simulink model "Buck_model"  (R2024a)
settings: Solver=odeN  StartTime=0.0  StopTime=35  MaxStep=Ts_motor  RelTol=1e-3  EnableMultiTasking=on
InitFcn:
  | load bldcData
model workspace (MAT data in the model file):
  encoderResolution = 2000
  hallOffset = '0.5'
  indexOffset = 850
  polePairs = '4'
undefined symbols (not defined in the file or in its folder): DiscIntNeverNeededParam, Hecate_speed, Ts_motor
libraries: nesl_utility x25, fl_lib x24, ee_lib x7, batteryecm_lib x1, spsPWMGeneratorDCDCLib x1, slpidlib x1, simulink x1
(part 2 of 2)

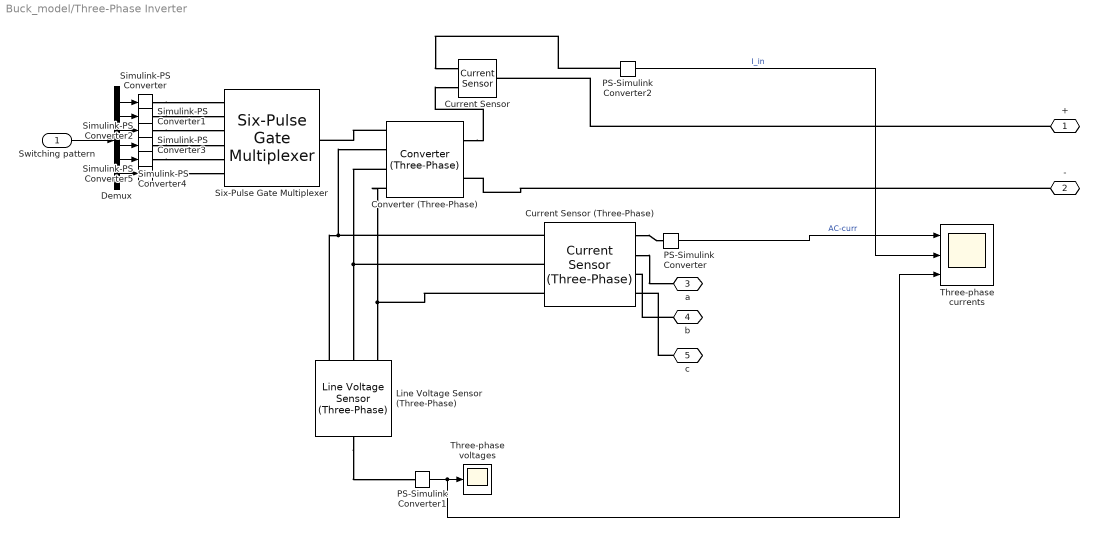
== system Buck_model/Three-Phase Inverter ==
  Switching pattern : Inport
  Converter (Three-Phase) : ee_lib/Semiconductors & Converters/Converters/Converter (Three-Phase)  port_option=ee.enum.threePhasePort.expanded  fidelity_option=ee.enum.converters.fidelity.detailed  device_type=ee.enum.converters.switchingdevice.mosfet  K=0  Vf=0.8 V  Ron=0.1 Ohm  Rds=0.001 Ohm  Goff=0.001 1/Ohm  Vgt=1 V  Vgt_off=-1 V  Ih=1 A  Vth=0.5 V  diode_param=ee.enum.converters.protectiondiode.nodynamics  diode_Vf=0.7 V  diode_Ron=0.001 Ohm  diode_Goff=1e-5 1/Ohm  diode_C=50 nF  diode_iRM=-235 A  diode_iF=300 A  diode_idot=-50 A/us  diode_trr_param=ee.enum.converters.diodetrr.trr_factor  diode_trr_factor=3  diode_trr=15 us  diode_Qrr=1500 s*uA  snubber_type=ee.enum.converters.snubber.include  Cs=1e-7 F  Rs=0.1 Ohm
      settings: InternalSimscapePortConfiguration="{\"Bottom\":[],\"Left\":[{\"id\":\"G\",\"label\":\"G\",\"type\":\"foundation.electrical.twelve_phase\"},{\"id\":\"a\",\"label\":\"a\",\"type\":\"foundation.electrical.electrical\"},{\"id\":\"b\",\"label\":\"b\",\"type\":\"foundation.electrical.electrical\"},{\"id\":\"c\",\"label\":\"c\",\"type\":\"foundation.electrical.electrical\"}],\"Right\":[{\"id\":\"p\",\"label\":\"+\",\"type\":\"foundation.electrical.electrical\"},{\"id\":\"n\",\"label\":\"-\",\"type\":\"foundation.electrical.electrical\"}],\"Top\":[]}"
  Current Sensor : fl_lib/Electrical/Electrical Sensors/Current Sensor
  Current Sensor (Three-Phase) : ee_lib/Sensors & Transducers/Current Sensor (Three-Phase)
      settings: InternalSimscapePortConfiguration="{\"Bottom\":[],\"Left\":[{\"id\":\"a1\",\"label\":\"a1\",\"type\":\"foundation.electrical.electrical\"},{\"id\":\"b1\",\"label\":\"b1\",\"type\":\"foundation.electrical.electrical\"},{\"id\":\"c1\",\"label\":\"c1\",\"type\":\"foundation.electrical.electrical\"}],\"Right\":[{\"id\":\"I_output\",\"label\":\"I\",\"type\":\"output\"},{\"id\":\"a2\",\"label\":\"a2\",\"type\":\"foundation.electrical.electrical\"},{\"id\":\"b2\",\"label\":\"b2\",\"type\":\"foundation.electrical.electrical\"},{\"id\":\"c2\",\"label\":\"c2\",\"type\":\"foundation.electrical.electrical\"}],\"Top\":[]}"
  Demux : Demux  Outputs=6
  Line Voltage Sensor (Three-Phase) : ee_lib/Sensors & Transducers/Line Voltage Sensor (Three-Phase)
      settings: InternalSimscapePortConfiguration="{\"Bottom\":[],\"Left\":[{\"id\":\"a\",\"label\":\"a\",\"type\":\"foundation.electrical.electrical\"},{\"id\":\"b\",\"label\":\"b\",\"type\":\"foundation.electrical.electrical\"},{\"id\":\"c\",\"label\":\"c\",\"type\":\"foundation.electrical.electrical\"}],\"Right\":[{\"id\":\"V_output\",\"label\":\"V\",\"type\":\"output\"}],\"Top\":[]}"
  PS-Simulink Converter : nesl_utility/PS-Simulink Converter  PhysicalDomain=network_engine_domain  SubClassName=ps_output  LeftPortType=input  RightPortType=output  PseudoPeriodic=off  Frequencies=[]  VectorFormat=1-D array  Unit=1  AffineConversion=off
  PS-Simulink Converter1 : nesl_utility/PS-Simulink Converter  PhysicalDomain=network_engine_domain  SubClassName=ps_output  LeftPortType=input  RightPortType=output  PseudoPeriodic=off  Frequencies=[]  VectorFormat=1-D array  Unit=1  AffineConversion=off
  PS-Simulink Converter2 : nesl_utility/PS-Simulink Converter  PhysicalDomain=network_engine_domain  SubClassName=ps_output  LeftPortType=input  RightPortType=output  PseudoPeriodic=off  Frequencies=[]  VectorFormat=1-D array  Unit=1  AffineConversion=off
  Simulink-PS Converter{,1..5} (6 alike) : nesl_utility/Simulink-PS Converter  PhysicalDomain=network_engine_domain  SubClassName=ps_input  LeftPortType=input  RightPortType=output  PseudoPeriodic=off  Frequencies=[]  NoiseDistribution=none  NoiseParameters=[]  Unit=1  AffineConversion=off  FilteringAndDerivatives=provide  SimscapeFilterOrder=1  InputFilterTimeConstant=0.001  UdotUserProvided=0
  Six-Pulse Gate Multiplexer : ee_lib/Semiconductors & Converters/Converters/Six-Pulse Gate Multiplexer  port_option=ee.enum.controlport.ps
  Three-phase currents : Scope  NumInputPorts=3
  Three-phase voltages : Scope
  + : PMIOPort  Side=Left
  - : PMIOPort  Port=2  Side=Left
  a : PMIOPort  Port=3  Side=Right
  b : PMIOPort  Port=4  Side=Right
  c : PMIOPort  Port=5  Side=Right
  wires:
  PS-Simulink Converter1/1 -> Three-phase currents/3, Three-phase voltages/1
  PS-Simulink Converter/1 -> Three-phase currents/1  "AC-curr"
  Switching pattern/1 -> Demux/1
  Demux/1 -> Simulink-PS Converter/1
  Demux/2 -> Simulink-PS Converter1/1
  Demux/3 -> Simulink-PS Converter2/1
  Demux/4 -> Simulink-PS Converter3/1
  Demux/5 -> Simulink-PS Converter4/1
  Demux/6 -> Simulink-PS Converter5/1
  PS-Simulink Converter2/1 -> Three-phase currents/2  "I_in"
  connections:
  Current Sensor (Three-Phase)/RConn1 -- PS-Simulink Converter/LConn1
  Simulink-PS Converter/RConn1 -- Six-Pulse Gate Multiplexer/LConn1
  Simulink-PS Converter1/RConn1 -- Six-Pulse Gate Multiplexer/LConn2
  Simulink-PS Converter2/RConn1 -- Six-Pulse Gate Multiplexer/LConn3
  Simulink-PS Converter3/RConn1 -- Six-Pulse Gate Multiplexer/LConn4
  Simulink-PS Converter4/RConn1 -- Six-Pulse Gate Multiplexer/LConn5
  Simulink-PS Converter5/RConn1 -- Six-Pulse Gate Multiplexer/LConn6
  Converter (Three-Phase)/LConn1 -- Six-Pulse Gate Multiplexer/RConn1
  Line Voltage Sensor (Three-Phase)/LConn1 -- Current Sensor (Three-Phase)/LConn1 -- Converter (Three-Phase)/LConn2
  Line Voltage Sensor (Three-Phase)/RConn1 -- PS-Simulink Converter1/LConn1
  Converter (Three-Phase)/LConn3 -- Current Sensor (Three-Phase)/LConn2 -- Line Voltage Sensor (Three-Phase)/LConn2
  Converter (Three-Phase)/LConn4 -- Current Sensor (Three-Phase)/LConn3 -- Line Voltage Sensor (Three-Phase)/LConn3
  Current Sensor (Three-Phase)/RConn2 -- a/RConn1
  b/RConn1 -- Current Sensor (Three-Phase)/RConn3
  c/RConn1 -- Current Sensor (Three-Phase)/RConn4
  -/RConn1 -- Converter (Three-Phase)/RConn2
  +/RConn1 -- Current Sensor/LConn1
  Converter (Three-Phase)/RConn1 -- Current Sensor/RConn2
  PS-Simulink Converter2/LConn1 -- Current Sensor/RConn1

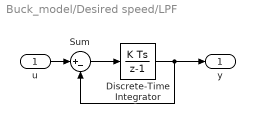
== system Buck_model/Desired speed/LPF ==
  u : Inport
  Discrete-Time Integrator : DiscreteIntegrator  gainval=20  SampleTime=Ts_motor  ICPrevOutput=DiscIntNeverNeededParam  ICPrevScaledInput=DiscIntNeverNeededParam
  Sum : Sum  Inputs=|+-
  y : Outport
  wires:
  Sum/1 -> Discrete-Time Integrator/1
  Discrete-Time Integrator/1 -> y/1, Sum/2
  u/1 -> Sum/1

== stateflow chart Buck_model/Test Assessment ==
  state SpeedLimit_0
    state step_1
    state step_2
      verify(speed >= 0.0001);
    (default) -> SpeedLimit_0.step_1
    SpeedLimit_0.step_1 -> SpeedLimit_0.step_2 : [
        | after(2, 'sec')
        | ]
  state SpeedLimit_170
    state Speed_Hecate
      verify(speed <=  170);
    (default) -> SpeedLimit_170.Speed_Hecate
  state SpeedLimit_HS
    state step_1
    state Speed_Hecate
      verify(speed <= Hecate_speed+ 0.5);
    state step_2
    state step_3
      verify(speed <= Hecate_speed+ 0.5);
    (default) -> SpeedLimit_HS.step_1
    SpeedLimit_HS.step_1 -> SpeedLimit_HS.Speed_Hecate : [
        | after(6, 'sec')
        | ]
    SpeedLimit_HS.Speed_Hecate -> SpeedLimit_HS.step_2 : [
        | after(4, 'sec')
        | ]
    SpeedLimit_HS.step_2 -> SpeedLimit_HS.step_3 : [
        | after(16, 'sec')
        | ]
    SpeedLimit_HS.step_3 -> SpeedLimit_HS.step_2 : [
        | after(4, 'sec')
        | ]
  state SpeedLimit_HS_subtest
    state step_1
    state Speed_Hecate
      verify(speed <= (Hecate_speed + 1));
    state step_2
    state step_3
      verify(speed <= (Hecate_speed + 1));
    (default) -> SpeedLimit_HS_subtest.step_1
    SpeedLimit_HS_subtest.step_1 -> SpeedLimit_HS_subtest.Speed_Hecate : [
        | after(6, 'sec')
        | ]
    SpeedLimit_HS_subtest.Speed_Hecate -> SpeedLimit_HS_subtest.step_2 : [
        | after(4, 'sec')
        | ]
    SpeedLimit_HS_subtest.step_2 -> SpeedLimit_HS_subtest.step_3 : [
        | after(16, 'sec')
        | ]
    SpeedLimit_HS_subtest.step_3 -> SpeedLimit_HS_subtest.step_2 : [
        | after(4, 'sec')
        | ]
  (default) -> SpeedLimit_0 [order 1] : [Active_Scenario_Index == 1]
  (default) -> SpeedLimit_170 [order 2] : [Active_Scenario_Index == 2]
  (default) -> SpeedLimit_HS [order 3] : [Active_Scenario_Index == 3]
  (default) -> SpeedLimit_HS_subtest [order 4] : {assert(Active_Scenario_Index == 4,'The value of Scenario Parameter ''Active_Scenario_Index'' is not valid. Use the index of the scenario to specify it.')}
  data: speed input; Active_Scenario_Index parameter =1; Hecate_speed parameter

== stateflow chart Buck_model/FitnessConverter_Hecate ==
  state step_1
    fitness_1 = Inf;
  state step_2
    fitness_1 = speed-(0.0001);
  (default) -> step_1
  step_1 -> step_2 : [after(2, 'sec')]
  data: speed input; Hecate_speed parameter; fitness_1 output

== stateflow chart Buck_model/Test Sequence  ==
  state Grafico_Scalino_1
    state step_1
      speed = 0;
    state step_2
      speed = Hecate_speed;
    (default) -> Grafico_Scalino_1.step_1
    Grafico_Scalino_1.step_1 -> Grafico_Scalino_1.step_2 : [
        | after(1,'sec')
        | ]
    Grafico_Scalino_1.step_2 -> Grafico_Scalino_1.step_1 : [
        | after(4,'sec')
        | ]
  state Grafico_Scalino_2
    state step_1
      speed = 85;
    state step_2
      speed = Hecate_speed;
    (default) -> Grafico_Scalino_2.step_1
    Grafico_Scalino_2.step_1 -> Grafico_Scalino_2.step_2 : [
        | after(1,'sec')
        | ]
    Grafico_Scalino_2.step_2 -> Grafico_Scalino_2.step_1 : [
        | after(4,'sec')
        | ]
  state Grafico_Scalino_3
    state step_1
      speed = 130;
    state step_2
      speed = Hecate_speed;
    (default) -> Grafico_Scalino_3.step_1
    Grafico_Scalino_3.step_1 -> Grafico_Scalino_3.step_2 : [
        | after(1,'sec')
        | ]
    Grafico_Scalino_3.step_2 -> Grafico_Scalino_3.step_1 : [
        | after(4,'sec')
        | ]
  state Grafico_DoppioTronco_1
    state step_1
      getSimulationTime()
      speed = 0 + (Hecate_speed - 0) / (5 - 0) * getSimulationTime();
    state step_2
      speed = Hecate_speed;
    state step_3
      speed = Hecate_speed + (0 - Hecate_speed) / (15 - 10) * (getSimulationTime - 10);
    state step_4
      speed = 0;
    state step_5
      speed = 0 + (Hecate_speed - 0) / (5 - 0) * (getSimulationTime() - 20);
    state step_6
      speed = Hecate_speed;
    state step_7
      speed = Hecate_speed + (0 - Hecate_speed) / (15 - 10) * (getSimulationTime - 30);
    (default) -> Grafico_DoppioTronco_1.step_1
    Grafico_DoppioTronco_1.step_1 -> Grafico_DoppioTronco_1.step_2 : [
        | after(5, 'sec')
        | ]
    Grafico_DoppioTronco_1.step_2 -> Grafico_DoppioTronco_1.step_3 : [
        | after(5, 'sec')
        | ]
    Grafico_DoppioTronco_1.step_3 -> Grafico_DoppioTronco_1.step_4 : [
        | after(5, 'sec')
        | ]
    Grafico_DoppioTronco_1.step_4 -> Grafico_DoppioTronco_1.step_5 : [
        | after(5, 'sec')
        | ]
    Grafico_DoppioTronco_1.step_5 -> Grafico_DoppioTronco_1.step_6 : [
        | after(5, 'sec')
        | ]
    Grafico_DoppioTronco_1.step_6 -> Grafico_DoppioTronco_1.step_7 : [
        | after(5, 'sec')
        | ]
  state Grafico_DoppioTronco_2
    state step_1
      getSimulationTime()
      speed = 85 + (Hecate_speed - 85) / (5 - 0) * getSimulationTime();
    state step_2
      speed = Hecate_speed;
    state step_3
      speed = Hecate_speed + (85 - Hecate_speed) / (15 - 10) * (getSimulationTime - 10);
    state step_4
      speed = 85;
    state step_5
      speed = 85 + (Hecate_speed - 85) / (5 - 0) * (getSimulationTime() - 20);
    state step_6
      speed = Hecate_speed;
    state step_7
      speed = Hecate_speed + (85 - Hecate_speed) / (15 - 10) * (getSimulationTime - 30);
    (default) -> Grafico_DoppioTronco_2.step_1
    Grafico_DoppioTronco_2.step_1 -> Grafico_DoppioTronco_2.step_2 : [
        | after(5, 'sec')
        | ]
    Grafico_DoppioTronco_2.step_2 -> Grafico_DoppioTronco_2.step_3 : [
        | after(5, 'sec')
        | ]
    Grafico_DoppioTronco_2.step_3 -> Grafico_DoppioTronco_2.step_4 : [
        | after(5, 'sec')
        | ]
    Grafico_DoppioTronco_2.step_4 -> Grafico_DoppioTronco_2.step_5 : [
        | after(5, 'sec')
        | ]
    Grafico_DoppioTronco_2.step_5 -> Grafico_DoppioTronco_2.step_6 : [
        | after(5, 'sec')
        | ]
    Grafico_DoppioTronco_2.step_6 -> Grafico_DoppioTronco_2.step_7 : [
        | after(5, 'sec')
        | ]
  state Grafico_DoppioTronco_3
    state step_1
      getSimulationTime()
      speed = 130 + (Hecate_speed - 130) / (5 - 0) * getSimulationTime();
    state step_2
      speed = Hecate_speed;
    state step_3
      speed = Hecate_speed + (130 - Hecate_speed) / (15 - 10) * (getSimulationTime - 10);
    state step_4
      speed = 130;
    state step_5
      speed = 130 + (Hecate_speed - 130) / (5 - 0) * (getSimulationTime() - 20);
    state step_6
      speed = Hecate_speed;
    state step_7
      speed = Hecate_speed + (130 - Hecate_speed) / (15 - 10) * (getSimulationTime - 30);
    (default) -> Grafico_DoppioTronco_3.step_1
    Grafico_DoppioTronco_3.step_1 -> Grafico_DoppioTronco_3.step_2 : [
        | after(5, 'sec')
        | ]
    Grafico_DoppioTronco_3.step_2 -> Grafico_DoppioTronco_3.step_3 : [
        | after(5, 'sec')
        | ]
    Grafico_DoppioTronco_3.step_3 -> Grafico_DoppioTronco_3.step_4 : [
        | after(5, 'sec')
        | ]
    Grafico_DoppioTronco_3.step_4 -> Grafico_DoppioTronco_3.step_5 : [
        | after(5, 'sec')
        | ]
    Grafico_DoppioTronco_3.step_5 -> Grafico_DoppioTronco_3.step_6 : [
        | after(5, 'sec')
        | ]
    Grafico_DoppioTronco_3.step_6 -> Grafico_DoppioTronco_3.step_7 : [
        | after(5, 'sec')
        | ]
  (default) -> Grafico_Scalino_1 [order 1] : [Active_Scenario_Index == 1]
  (default) -> Grafico_Scalino_2 [order 2] : [Active_Scenario_Index == 2]
  (default) -> Grafico_Scalino_3 [order 3] : [Active_Scenario_Index == 3]
  (default) -> Grafico_DoppioTronco_1 [order 4] : [Active_Scenario_Index == 4]
  (default) -> Grafico_DoppioTronco_2 [order 5] : [Active_Scenario_Index == 5]
  (default) -> Grafico_DoppioTronco_3 [order 6] : {assert(Active_Scenario_Index == 6,'The value of Scenario Parameter ''Active_Scenario_Index'' is not valid. Use the index of the scenario to specify it.')}
  data: speed output; Active_Scenario_Index parameter =1; Hecate_speed parameter
